simulink model "prog1_mod"  (R2015b)
settings: Solver=ode113  StartTime=0.0  StopTime=10.0  FixedStep=0.0000001  RelTol=1e-9  AbsTol=1e-9
values from neighbouring files (symbols this model uses):
  g = 2000    [prog1.m]
  OM1 = 200*pi    (= 628.318530718)    [prog1.m]
  OM2 = 2000*pi    (= 6283.18530718)    [prog1.m]
  Zet1 = 0.0796    [prog1.m]
  Zet2 = 0.05    [prog1.m]
libraries: simulink x1
settings Model: Creator=zap  LastModifiedBy=zap

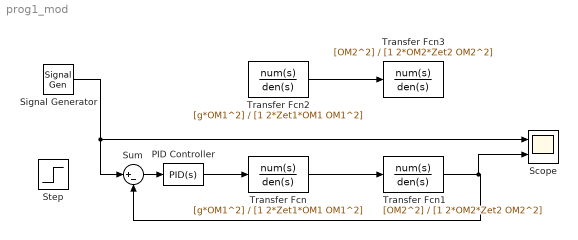
== system prog1_mod ==
  PID Controller : simulink/Continuous/PID Controller  Controller=PID  TimeDomain=Continuous-time  SampleTime=-1  IntegratorMethod=Forward Euler  FilterMethod=Forward Euler  Form=Parallel  UseFilter=on  ControllerParametersSource=internal  P=0.003  I=0.0  D=0  N=100  InitialConditionSource=internal  InitialConditionForIntegrator=0  InitialConditionForFilter=0  ExternalReset=none  LimitOutput=off  UpperSaturationLimit=inf  LowerSaturationLimit=-inf  LinearizeAsGain=on  AntiWindupMode=none  Kb=1  TrackingMode=off  Kt=1  PParamMin=[]  PParamMax=[]  IParamMin=[]  IParamMax=[]  DParamMin=[]  DParamMax=[]  NParamMin=[]  NParamMax=[]  KbParamMin=[]  KbParamMax=[]  KtParamMin=[]  KtParamMax=[]  POutMin=[]  POutMax=[]  IOutMin=[]  IOutMax=[]  DOutMin=[]  DOutMax=[]  NOutMin=[]  NOutMax=[]  KbOutMin=[]  KbOutMax=[]  KtOutMin=[]  KtOutMax=[]  IntegratorOutMin=[]  IntegratorOutMax=[]  FilterOutMin=[]  FilterOutMax=[]  SumOutMin=[]  SumOutMax=[]  SumI1OutMin=[]  SumI1OutMax=[]  SumI2OutMin=[]  SumI2OutMax=[]  SumI3OutMin=[]  SumI3OutMax=[]  SumDOutMin=[]  SumDOutMax=[]  SaturationOutMin=[]  SaturationOutMax=[]  IntegratorContinuousStateAttributes=''  IntegratorStateMustResolveToSignalObject=off  IntegratorRTWStateStorageClass=Auto  FilterContinuousStateAttributes=''  FilterStateMustResolveToSignalObject=off  FilterRTWStateStorageClass=Auto  DifferentiatorICPrevScaledInput=0  DifferentiatorOutMin=[]  DifferentiatorOutMax=[]
  Scope : Scope  NumInputPorts=2
  Signal Generator : SignalGenerator  WaveForm=square  Frequency=3  Units=rad/sec
  Step : Step  Time=0  SampleTime=0
  Sum : Sum  Inputs=|+-
  Transfer Fcn : TransferFcn  Numerator=[g*OM1^2]  Denominator=[1 2*Zet1*OM1 OM1^2]  AbsoluteTolerance=10^-12
  Transfer Fcn1 : TransferFcn  Numerator=[OM2^2]  Denominator=[1 2*OM2*Zet2 OM2^2]  AbsoluteTolerance=10^-12
  Transfer Fcn2 : TransferFcn  Numerator=[g*OM1^2]  Denominator=[1 2*Zet1*OM1 OM1^2]  AbsoluteTolerance=10^-12
  Transfer Fcn3 : TransferFcn  Numerator=[OM2^2]  Denominator=[1 2*OM2*Zet2 OM2^2]  AbsoluteTolerance=10^-12
  wires:
  Transfer Fcn/1 -> Transfer Fcn1/1
  Transfer Fcn1/1 -> Scope/2, Sum/2
  Sum/1 -> PID Controller/1
  PID Controller/1 -> Transfer Fcn/1
  Transfer Fcn2/1 -> Transfer Fcn3/1
  Signal Generator/1 -> Scope/1, Sum/1
